simulink model "laser_simulink"  (R2021a)
settings: Solver=VariableStepAuto  StartTime=0.0  StopTime=10.0  RelTol=1e-3
settings Model: Creator=USER  LastModifiedBy=USER

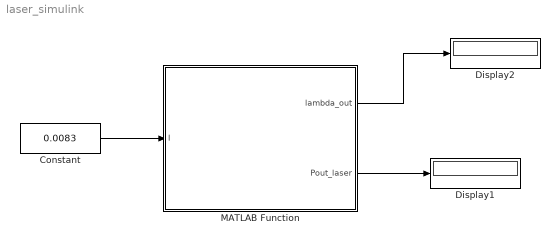
== system laser_simulink ==
  Constant : Constant  Value=0.0083
  Display1 : Display
  Display2 : Display
  MATLAB Function : MATLAB Function  TreatAsAtomicUnit=on
  wires:
  Constant/1 -> MATLAB Function/1(I)
  MATLAB Function/2(Pout_laser) -> Display1/1
  MATLAB Function/1(lambda_out) -> Display2/1

== matlab function laser_simulink/MATLAB Function ==
  data: I input; lambda_out output; Pout_laser output
function [lambda_out,Pout_laser] = laser_func(I)
% This code is intended to model a semiconductor laser

%% parameter definition

N0 = 6.5e23;
a0 = 3.13e-20;
a_bar = 1.2;
lambda_0 = 1.575e-6;
b0 = 3.17e-26*1e-6;
b1 = 0;
lambda_z0 = 1.625e-6;
z0 = -2.5e-27*1e-6;
lambda_in = 0;
Pout_laser = 0;
%% plotting for discrete concentration values

% N = [3 2.5 2 1]*1e24;
% lambda = [1.45:0.01:1.65]*1e-6;
% hw = 1243./(lambda*1e9);
% 
% gp = zeros(1,length(N));
% lambda_p = zeros(1,length(N));
% lambda_z = zeros(1,length(N));
% cn = zeros(1,length(N));
% dn = zeros(1,length(N));
% gm = zeros(length(lambda), length(N));
% 
% for j=1:length(lambda)
%     for i=1:length(N)
% 
%         gp(i) = a0*(N(i)-N0) + a0*a_bar*N0*exp(-N(i)/N0);
%         lambda_p(i) = lambda_0 - (b0*(N(i)-N0) + b1*((N(i)-N0)^2));
%         lambda_z(i) = lambda_z0 - z0*(N(i)-N0);
% 
%         cn(i) = 3*gp(i)/((lambda_z(i)-lambda_p(i))^2);
%         dn(i) = 2*gp(i)/((lambda_z(i)-lambda_p(i))^3);
% 
%         if lambda(j)<lambda_z(i)
%             gm(j,i) = cn(i)*((lambda(j) - lambda_z(i)).^2) + ...
%                 dn(i)*((lambda(j) - lambda_z(i)).^3);
%         end
%     end
% end

% figure()
% for i=1:length(N)
%     plot(lambda, gm(:,i));
%     hold on
% end
% xlabel('Lambda(um)')
% ylabel('gm')
% legend('3', '2.5', '2', '1')
% title('gm vs lambda for differnet conc.')
%% plotting for continuous concentration values

N = [0.1:0.01:3]*1e24;
lambda = [1.45:0.01:1.65]*1e-6;
hw = 1243./(lambda*1e9);

gp = zeros(1,length(N));
lambda_p = zeros(1,length(N));
lambda_z = zeros(1,length(N));
cn = zeros(1,length(N));
dn = zeros(1,length(N));
gm = zeros(length(N), length(lambda));
gpeak = zeros(1,length(N));

for i=1:length(N)
    for j=1:length(lambda)

        gp(i) = a0*(N(i)-N0) + a0*a_bar*N0*exp(-N(i)/N0);
        lambda_p(i) = lambda_0 - (b0*(N(i)-N0) + b1*((N(i)-N0)^2));
        lambda_z(i) = lambda_z0 - z0*(N(i)-N0);

        cn(i) = 3*gp(i)/((lambda_z(i)-lambda_p(i))^2);
        dn(i) = 2*gp(i)/((lambda_z(i)-lambda_p(i))^3);

        if lambda(j)<lambda_z(i)
            gm(i,j) = cn(i)*((lambda(j) - lambda_z(i)).^2) + ...
                dn(i)*((lambda(j) - lambda_z(i)).^3);
        end
    end

    gpeak(i) = max(gm(i,:));

end
% 
% figure()
% plot(N,gpeak);
% xlabel('N')
% ylabel('gpeak')
% title('geak vs conc.')
%% parameter definition from book example for semiconductor laser

L = 100e-6;
W = 3e-6;
d = 0.15e-6;
gamma = 2500; %loss coefficient per meter
nr = 3.491; %In0.6 Ga0.4 As0.85 P0.15 http://www.ioffe.ru/SVA/NSM/Semicond/GaInAsP/optic.html
R = ((nr-1)^2)/((nr+1)^2);
B = 2e-16; %exercise 4.30
e = 1.6e-19;
c = 3e8;
h = 6.626e-34;


%% calculating loss
confinement = 1;
alpha_t = gamma + (1/(2*L))*log(1/(R*R)); %total loss
gth = alpha_t/confinement;
gth_arr = gth*ones(1,length(N));
% plot(N,gpeak);
% hold on
% plot(N, gth_arr);
err = gpeak - gth_arr;
tolerance = 120;
index = find(abs(err)<tolerance);
nth = N(index); %threshold electron conc

%% plot allowed modes on the same plot as optical gain vs lambda
% figure()
% plot(lambda, gm(index,:))
% %lambda(find(max(gm(index,:))))
% hold on
% line([lambda(1) lambda(end)], [gth gth], 'Color', [0 0 0], 'LineWidth', 2);
% xlabel('Lambda(um)')
% ylabel('gm')
% title('gm vs lambda art threshold electron conc.')
max_index = find( gm(index,:) == max(gm(index,:)) );
lambda_in = lambda(max_index);

%% radiative lifetime calculation

tau_r = 1/(B*nth);

%% Threshold current density

Jth = nth*e*d/tau_r;
Ith = W*L*Jth;

%% Photon cavity lifetime

tau_ph = nr/(c*alpha_t);

%% Output Power

%I = 7.4e-3; %from solar cell
%lambda_in = 1500e-9; %from figure 4.48
Pout_slope = (h*c*c*tau_ph*(1-R)/(2*e*nr*lambda_in*L));
Pout = Pout_slope*(I-Ith);

lambda_out = lambda_in;
Pout_laser = Pout;
end
